simulink model "motor"  (R2022b)
settings: Solver=VariableStepAuto  StartTime=0.0  StopTime=0.1  MaxStep=1e-3  RelTol=1e-3
settings Model: Creator=Dell  LastModifiedBy=Dell

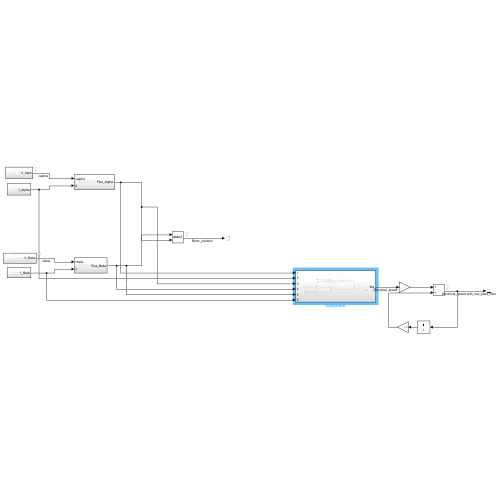
[thumbnail: Simulink's stored preview of the top-level diagram]
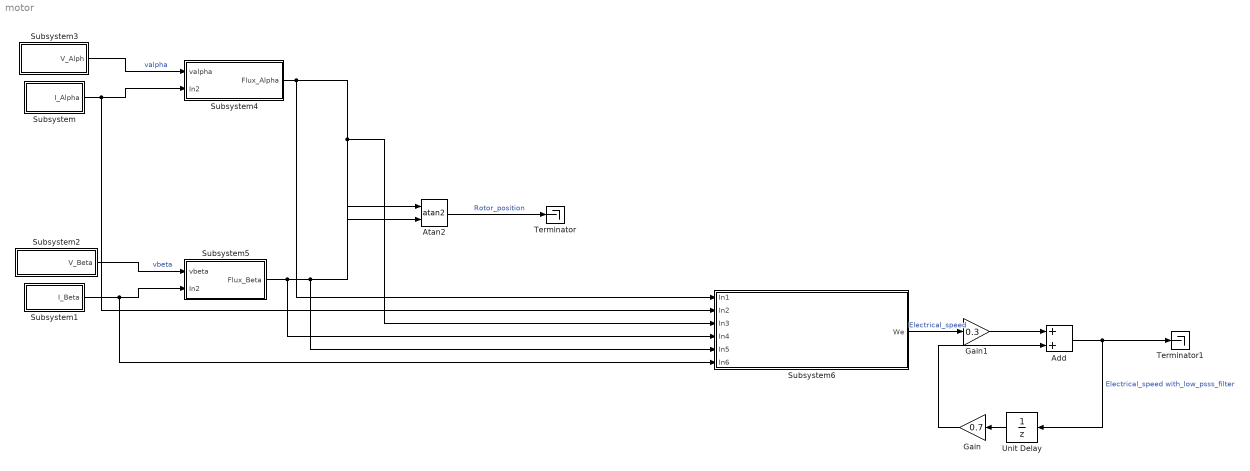
== system motor ==
  Add : Sum
  Atan2 : Trigonometry  Operator=atan2
  Gain : Gain  Gain=0.7
  Gain1 : Gain  Gain=0.3
  Subsystem : Subsystem
  Subsystem1 : Subsystem
  Subsystem2 : Subsystem
  Subsystem3 : Subsystem
  Subsystem4 : Subsystem
  Subsystem5 : Subsystem
  Subsystem6 : Subsystem
  Terminator : Terminator
  Terminator1 : Terminator
  Unit Delay : UnitDelay  SampleTime=-1  HasFrameUpgradeWarning=on
  wires:
  Atan2/1 -> Terminator/1  "Rotor_position"
  Subsystem3/1(V_Alph) -> Subsystem4/1(valpha)  "valpha"
  Subsystem/1(I_Alpha) -> Subsystem6/2(In2), Subsystem4/2(In2)
  Subsystem4/1(Flux_Alpha) -> Subsystem6/1(In1), Subsystem6/3(In3), Atan2/2
  Subsystem2/1(V_Beta) -> Subsystem5/1(vbeta)  "vbeta"
  Subsystem1/1(I_Beta) -> Subsystem6/6(In6), Subsystem5/2(In2)
  Subsystem5/1(Flux_Beta) -> Subsystem6/4(In4), Subsystem6/5(In5), Atan2/1
  Subsystem6/1(We) -> Gain1/1  "Electrical_speed"
  Unit Delay/1 -> Gain/1
  Gain/1 -> Add/2
  Gain1/1 -> Add/1
  Add/1 -> Unit Delay/1, Terminator1/1  "Electrical_speed with_low_psss_filter"

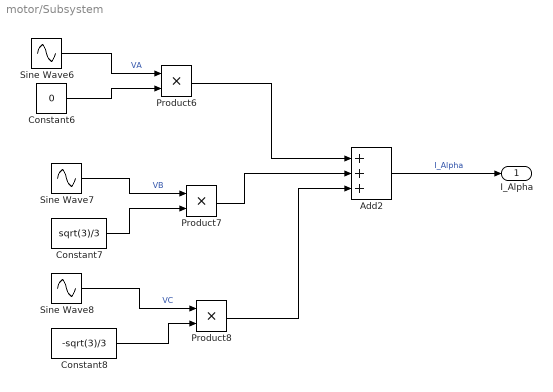
== system motor/Subsystem ==
  Add2 : Sum  Inputs=+++
  Constant6 : Constant  Value=0
  Constant7 : Constant  Value=sqrt(3)/3
  Constant8 : Constant  Value=-sqrt(3)/3
  Product6 : Product
  Product7 : Product
  Product8 : Product
  Sine Wave6 : Sin  Amplitude=2  Frequency=300  SampleTime=0
  Sine Wave7 : Sin  Amplitude=2  Frequency=300  Phase=(2/3)*pi  SampleTime=0
  Sine Wave8 : Sin  Amplitude=2  Frequency=300  Phase=(4/3)*pi  SampleTime=0
  I_Alpha : Outport
  wires:
  Constant8/1 -> Product8/2
  Product7/1 -> Add2/2
  Sine Wave6/1 -> Product6/1  "VA"
  Sine Wave8/1 -> Product8/1  "VC"
  Constant7/1 -> Product7/2
  Constant6/1 -> Product6/2
  Add2/1 -> I_Alpha/1  "I_Alpha"
  Sine Wave7/1 -> Product7/1  "VB"
  Product8/1 -> Add2/3
  Product6/1 -> Add2/1

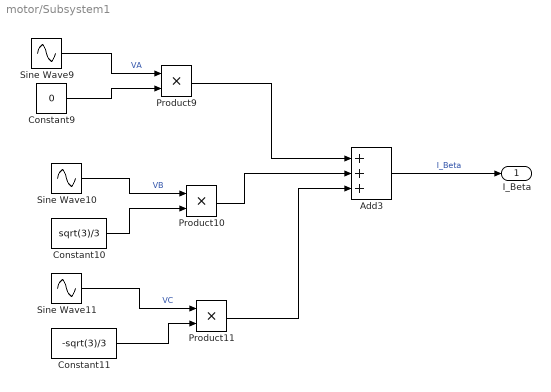
== system motor/Subsystem1 ==
  Add3 : Sum  Inputs=+++
  Constant10 : Constant  Value=sqrt(3)/3
  Constant11 : Constant  Value=-sqrt(3)/3
  Constant9 : Constant  Value=0
  Product10 : Product
  Product11 : Product
  Product9 : Product
  Sine Wave10 : Sin  Amplitude=2  Frequency=300  Phase=(2/3)*pi  SampleTime=0
  Sine Wave11 : Sin  Amplitude=2  Frequency=300  Phase=(4/3)*pi  SampleTime=0
  Sine Wave9 : Sin  Amplitude=2  Frequency=300  SampleTime=0
  I_Beta : Outport
  wires:
  Sine Wave10/1 -> Product10/1  "VB"
  Sine Wave9/1 -> Product9/1  "VA"
  Product9/1 -> Add3/1
  Constant11/1 -> Product11/2
  Constant10/1 -> Product10/2
  Constant9/1 -> Product9/2
  Sine Wave11/1 -> Product11/1  "VC"
  Product10/1 -> Add3/2
  Product11/1 -> Add3/3
  Add3/1 -> I_Beta/1  "I_Beta"

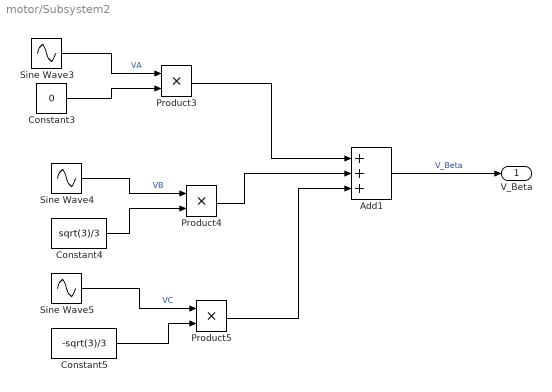
== system motor/Subsystem2 ==
  Add1 : Sum  Inputs=+++
  Constant3 : Constant  Value=0
  Constant4 : Constant  Value=sqrt(3)/3
  Constant5 : Constant  Value=-sqrt(3)/3
  Product3 : Product
  Product4 : Product
  Product5 : Product
  Sine Wave3 : Sin  Amplitude=12  Frequency=300  SampleTime=0
  Sine Wave4 : Sin  Amplitude=12  Frequency=300  Phase=(2/3)*pi  SampleTime=0
  Sine Wave5 : Sin  Amplitude=12  Frequency=300  Phase=(4/3)*pi  SampleTime=0
  V_Beta : Outport
  wires:
  Product4/1 -> Add1/2
  Product5/1 -> Add1/3
  Constant5/1 -> Product5/2
  Product3/1 -> Add1/1
  Constant3/1 -> Product3/2
  Sine Wave3/1 -> Product3/1  "VA"
  Sine Wave5/1 -> Product5/1  "VC"
  Constant4/1 -> Product4/2
  Sine Wave4/1 -> Product4/1  "VB"
  Add1/1 -> V_Beta/1  "V_Beta"

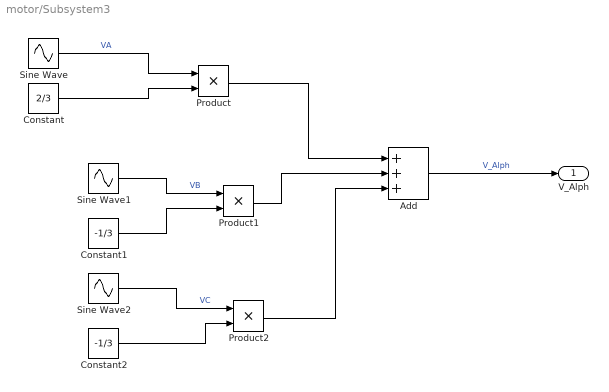
== system motor/Subsystem3 ==
  Add : Sum  Inputs=+++
  Constant : Constant  Value=2/3
  Constant1 : Constant  Value=-1/3
  Constant2 : Constant  Value=-1/3
  Product : Product
  Product1 : Product
  Product2 : Product
  Sine Wave : Sin  Amplitude=12  Frequency=300  SampleTime=0
  Sine Wave1 : Sin  Amplitude=12  Frequency=300  Phase=(2/3)*pi  SampleTime=0
  Sine Wave2 : Sin  Amplitude=12  Frequency=300  Phase=(4/3)*pi  SampleTime=0
  V_Alph : Outport
  wires:
  Product2/1 -> Add/3
  Product1/1 -> Add/2
  Constant2/1 -> Product2/2
  Product/1 -> Add/1
  Sine Wave/1 -> Product/1  "VA"
  Constant/1 -> Product/2
  Constant1/1 -> Product1/2
  Add/1 -> V_Alph/1  "V_Alph"
  Sine Wave1/1 -> Product1/1  "VB"
  Sine Wave2/1 -> Product2/1  "VC"

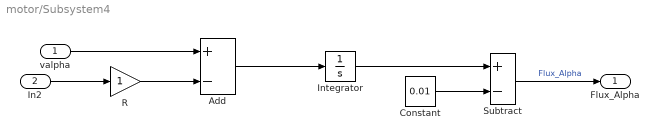
== system motor/Subsystem4 ==
  valpha : Inport
  In2 : Inport  Port=2
  Add : Sum  Inputs=+-
  Constant : Constant  Value=0.01
  Integrator : Integrator
  R : Gain
  Subtract : Sum  Inputs=+-
  Flux_Alpha : Outport
  wires:
  In2/1 -> R/1
  Constant/1 -> Subtract/2
  Add/1 -> Integrator/1
  valpha/1 -> Add/1
  Integrator/1 -> Subtract/1
  R/1 -> Add/2
  Subtract/1 -> Flux_Alpha/1  "Flux_Alpha"

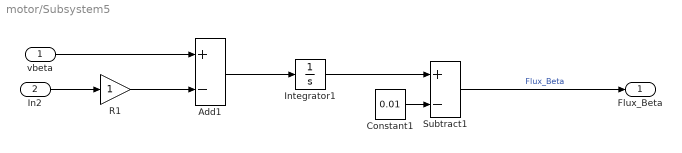
== system motor/Subsystem5 ==
  vbeta : Inport
  In2 : Inport  Port=2
  Add1 : Sum  Inputs=+-
  Constant1 : Constant  Value=0.01
  Integrator1 : Integrator
  R1 : Gain
  Subtract1 : Sum  Inputs=+-
  Flux_Beta : Outport
  wires:
  R1/1 -> Add1/2
  Add1/1 -> Integrator1/1
  Constant1/1 -> Subtract1/2
  Integrator1/1 -> Subtract1/1
  vbeta/1 -> Add1/1
  Subtract1/1 -> Flux_Beta/1  "Flux_Beta"
  In2/1 -> R1/1

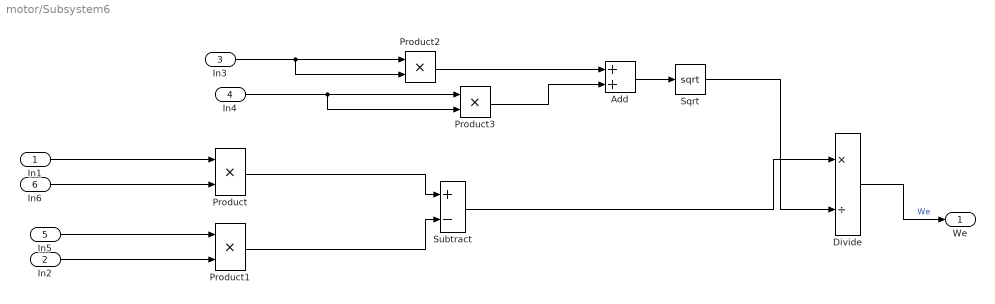
== system motor/Subsystem6 ==
  In1 : Inport
  In2 : Inport  Port=2
  In3 : Inport  Port=3
  In4 : Inport  Port=4
  In5 : Inport  Port=5
  In6 : Inport  Port=6
  Add : Sum
  Divide : Product  Inputs=*/
  Product{,1..3} (4 alike) : Product
  Sqrt : Sqrt
  Subtract : Sum  Inputs=+-
  We : Outport
  wires:
  Subtract/1 -> Divide/1
  Sqrt/1 -> Divide/2
  In1/1 -> Product/1
  In4/1 -> Product3/2, Product3/1
  Add/1 -> Sqrt/1
  Product2/1 -> Add/1
  In3/1 -> Product2/2, Product2/1
  Product3/1 -> Add/2
  Product1/1 -> Subtract/2
  Product/1 -> Subtract/1
  In6/1 -> Product/2
  In2/1 -> Product1/2
  Divide/1 -> We/1  "We"
  In5/1 -> Product1/1
